simulink model "Wind_turbine_model_L"  (R2020a)
settings: Solver=daessc  StartTime=0.0  StopTime=70  RelTol=1e-3
model workspace (MAT data in the model file):
  Tw = Simulink.Parameter
  Tw.Value = [0; 0; 24.07; 18.74; 14.42; 10.93; 8.08; 5.74; 5.8; 4.17; 2.78; 1.59; 0.56; -0.34; -1.13; -1.83; -2.46; -3.02; -3.52; -3.98; -4.39; -3.77; -4.12; -4.43; -4.73]
  Tw.DataType = 'auto'
  Tw.Dimensions = [25 1]
  c = Simulink.Parameter
  c.Value = [3.65; 4.43; 4.56; 4.36; 4.03; 3.68; 3.35; 3.05; 2.79; 2.56; 2.37; 2.19; 2.04; 1.91; 1.79; 1.68; 1.59; 1.5; 1.43; 1.36; 1.29; 1.24; 1.18; 1.14; 1.09]
  c.DataType = 'auto'
  c.Dimensions = [25 1]
  r = Simulink.Parameter
  r.Value = [1.8; 3.6; 5.4; 7.2; 9; 10.8; 12.6; 14.4; 16.2; 18; 19.8; 21.6; 23.4; 25.2; 27; 28.8; 30.6; 32.4; 34.2; 36; 37.8; 39.6; 41.4; 43.2; 45]
  r.DataType = 'auto'
  r.Dimensions = [25 1]
values from neighbouring files (symbols this model uses):
  a1 = 0.5176    [data.mat]
  a2 = 116    [data.mat]
  a3 = 0.4    [data.mat]
  a4 = 5    [data.mat]
  a5 = 21    [data.mat]
  a6 = 0.0068    [data.mat]
  a7 = 0.09    [data.mat]
  a8 = 0.035    [data.mat]
  Ad = 6031.85789489    [data.mat]
  D = 1e-3    (= 0.001)    [Generator_specs.m]
  denp = den_P    [Wind_Turbine_Pitch.m]    (also in data.mat = [91260000000000 145900000000000 1.431e+17 7.554e+15 2.279e+1)
  dent = den_P    [Wind_Turbine_Pitch.m]    (also in data.mat = [91260000000000 145900000000000 1.431e+17 7.554e+15 2.279e+1)
  f = 50    [Generator_specs.m]
  Fs = Vs*sqrt(2/3)/(2*pi*f)    [Generator_specs.m]
  fsw = 4e3    (= 4000)    [Generator_specs.m]
  J = 127/2    (= 63.5)    [Generator_specs.m]
  ki_id = (wn1^2)*Lr*sigma    (= 491.599501999)    [Generator_specs.m]
  ki_n = ((wnn^2)*J)/p    (= 203200)    [Generator_specs.m]
  Kopt = ((0.5*ro*pi*(Radius^5)*cp_max)/(lambda_opt^3))    (= 227539.221001)    [Generator_specs.m]
  kp_id = (2*wn1*sigma*Lr)-Rr    (= 0.5771)    [Generator_specs.m]
  kp_n = (2*wnn*J)/p    (= 5080)    [Generator_specs.m]
  Lm = 2.5e-3    (= 0.0025)    [Generator_specs.m]
  Lr = Lm + Lsi    (= 0.002587)    [Generator_specs.m]
  Ls = Lm + Lsi    (= 0.002587)    [Generator_specs.m]
  Lsi = 0.087e-3    (= 8.7e-05)    [Generator_specs.m]
  N = 100    [Generator_specs.m]
  nump = num_P    [Wind_Turbine_Pitch.m]    (also in data.mat = [16590000 26450000 25540000000 6335000000 3680000000000])
  numt = num_T    [Wind_Turbine_Pitch.m]    (also in data.mat = [-75000000 -527900000000 -306700000000000])
  p = 2    [Generator_specs.m]
  Ps = 2e6    (= 2000000)    [Generator_specs.m]
  Rr = 2.9e-3    (= 0.0029)    [Generator_specs.m]
  Rs = 2.6e-3    (= 0.0026)    [Generator_specs.m]
  s = tf('s')    [Wind_Turbine_Pitch.m]
  sigma = 1 - Lm^2/(Ls*Lr)    (= 0.0661284179513)    [Generator_specs.m]    (also in data.mat = 0.075)
  Tem = 12732    [Generator_specs.m]
  Tgd_max = 14000    [Wind_Turbine_Pitch.m]    (also in data.mat)
  Tie = 1    [data.mat]
  Tiu = 10000    [data.mat]
  Tix = 1    [data.mat]
  Tpe = 1    [data.mat]
  Tpu = 10000    [data.mat]
  Tpx = 10000    [data.mat]
  Ts = 1/fsw/50    (= 5e-06)    [Generator_specs.m]
  Vbus = Vr_stator*sqrt(2)    [Generator_specs.m]
  Vs = 690    [Generator_specs.m]
  WT_Params =     [data.mat]
undefined symbols (not defined in the file or in its folder): DiscIntNeverNeededParam, sigbuilder_block, X, Y, Z
libraries: sm_lib x21, fl_lib x18, nesl_utility x18, powerlib x8, sdl_lib x3, powerlib_meascontrol x1
(part 1 of 3)
settings Model: Creator=param  LastModifiedBy=param
settings SolverCC: ZeroCrossControl=DisableAll  ZeroCrossAlgorithm=Adaptive
settings ModelReferenceCC: EnableParallelModelReferenceBuilds=on  ModelReferenceMinAlgLoopOccurrences=on

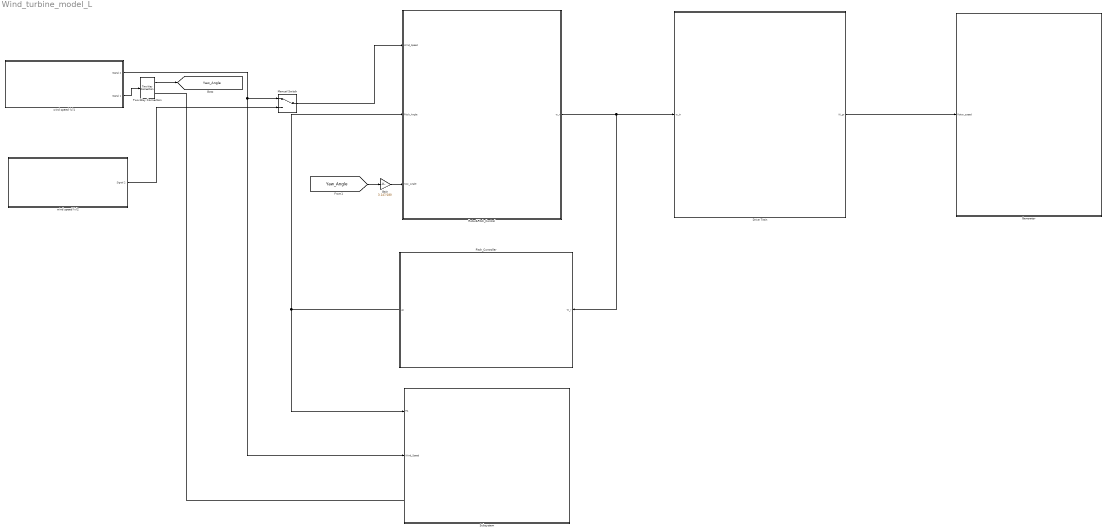
== system Wind_turbine_model_L ==
  Drive Train : Subsystem
  Gain : Gain  Gain=3.147/180
  Generator : Subsystem
  Manual Switch : ManualSwitch
  Pitch_Controller : Subsystem
  Rotor&Pitch_Control : Subsystem
  Subsystem : Subsystem
  Two-Way Connection : TwoWayConnection
  wind speed (v)1 : Subsystem  Tag=STV Subsys  LoadFcn=sigbuilder_block('load');  StartFcn=sigbuilder_block('start');  StopFcn=sigbuilder_block('stop');  ClipboardFcn=sigbuilder_block('clipboard');  mask(Sigbuilder block){tuvar=[0:10]}
      mask help: Simulink:masks:SigbuilderBlock_MD
      mask init:
      | if ~strcmp(get_param(bdroot(gcbh),'SimulationStatus'),'stopped') tuvar = sigbuilder_block('maskInit'); end
      settings: CopyFcn=sigbuilder_block('copy');  DeleteFcn=sigbuilder_block('delete');  ModelCloseFcn=sigbuilder_block('modelClose');  PreSaveFcn=sigbuilder_block('preSave');  PauseFcn=sigbuilder_block('pause');  ContinueFcn=sigbuilder_block('continue');  NameChangeFcn=sigbuilder_block('namechange');  OpenFcn=sigbuilder_block('open',[6 0 1012.5 477.75 ]);  CloseFcn=sigbuilder_block('close');
      mask Display: plot(0, 0, 100, 100,[2, 2, 32, 32, 2], [68, 8, 8, 68, 68],[32, 2], [38, 38], [32, 19, 2],[53, 60, 44], [32, 17, 17, 2],[16, 16, 31, 31]);txt = getActiveGroup(gcbh);text(2, 100, txt,'verticalAlignment', 'top');
  wind speed (v)2 : Subsystem  Tag=STV Subsys  LoadFcn=sigbuilder_block('load');  StartFcn=sigbuilder_block('start');  StopFcn=sigbuilder_block('stop');  ClipboardFcn=sigbuilder_block('clipboard');  mask(Sigbuilder block){tuvar=[0:10]}
      mask help: Simulink:masks:SigbuilderBlock_MD
      mask init:
      | if ~strcmp(get_param(bdroot(gcbh),'SimulationStatus'),'stopped') tuvar = sigbuilder_block('maskInit'); end
      settings: CopyFcn=sigbuilder_block('copy');  DeleteFcn=sigbuilder_block('delete');  ModelCloseFcn=sigbuilder_block('modelClose');  PreSaveFcn=sigbuilder_block('preSave');  PauseFcn=sigbuilder_block('pause');  ContinueFcn=sigbuilder_block('continue');  NameChangeFcn=sigbuilder_block('namechange');  OpenFcn=sigbuilder_block('open',[289.8 114 442.2 307.8 ]);  CloseFcn=sigbuilder_block('close');
      mask Display: plot(0, 0, 100, 100,[2, 2, 32, 32, 2], [68, 8, 8, 68, 68],[32, 2], [38, 38], [32, 19, 2],[53, 60, 44], [32, 17, 17, 2],[16, 16, 31, 31]);txt = getActiveGroup(gcbh);text(2, 100, txt,'verticalAlignment', 'top');
  tag scope: Yaw_Angle=global
  wires:
  Drive Train/1(W_gr) -> Generator/1(Rotor_speed)
  Rotor&Pitch_Control/1(w_r) -> Pitch_Controller/1(W_r), Drive Train/1(w_tr)
  wind speed (v)2/1(Signal 2) -> Manual Switch/2
  Manual Switch/1 -> Rotor&Pitch_Control/1(Wind_Speed)
  wind speed (v)1/1(Signal 2) -> Manual Switch/1, Subsystem/2(Wind_Speed)
  wind speed (v)1/2(Signal 1) -> Two-Way Connection/1
  [Yaw_Angle] -> Gain/1
  Two-Way Connection/1 -> [Yaw_Angle]
  Gain/1 -> Rotor&Pitch_Control/3(Yaw_Angle)
  Pitch_Controller/1(up) -> Subsystem/1(PA), Rotor&Pitch_Control/2(Pitch_Angle)
  connections:
  Subsystem/LConn1 -- Two-Way Connection/RConn1

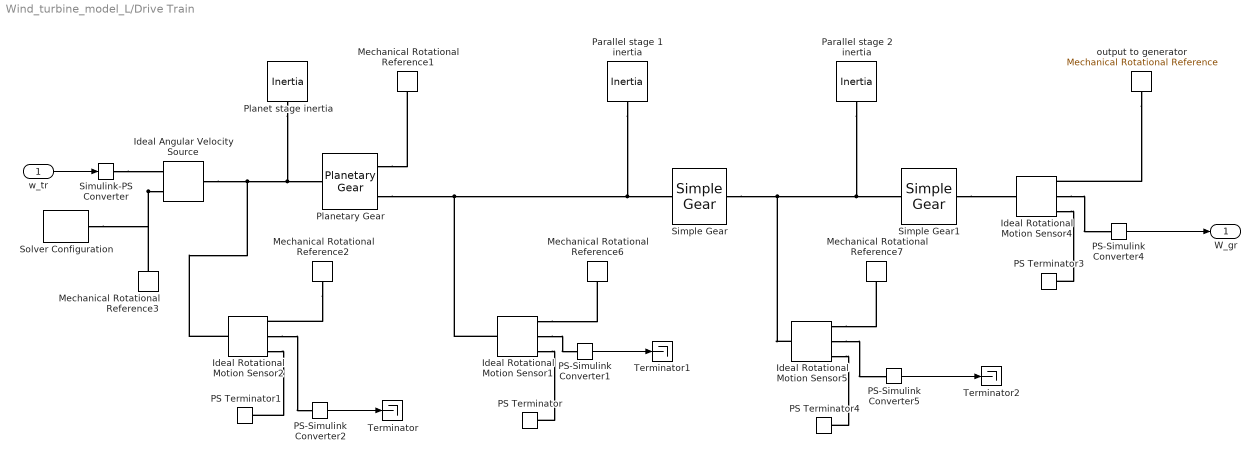
== system Wind_turbine_model_L/Drive Train ==
  w_tr : Inport
  Ideal Angular Velocity Source : fl_lib/Mechanical/Mechanical Sources/Ideal Angular Velocity Source
  Ideal Rotational Motion Sensor{1..2,4..5} (4 alike) : fl_lib/Mechanical/Mechanical Sensors/Ideal Rotational Motion Sensor  wrap_angle=simscape.enum.onoff.off  offset=0 rad
  Mechanical Rotational Reference{1..3,6..7} (5 alike) : fl_lib/Mechanical/Rotational Elements/Mechanical Rotational Reference
  PS Terminator{,1,3..4} (4 alike) : fl_lib/Physical Signals/Sinks/PS Terminator
  PS-Simulink Converter{1..2,4..5} (4 alike) : nesl_utility/PS-Simulink Converter  PhysicalDomain=network_engine_domain  SubClassName=ps_output  LeftPortType=input  RightPortType=output  PseudoPeriodic=off  Frequencies=[]  Unit=inherit  AffineConversion=off
  Parallel stage 1 inertia : fl_lib/Mechanical/Rotational Elements/Inertia  inertia=100 kg*m^2  w_specify=off  w_priority=High  w=0 rad/s  w_nominal_specify=off  w_nominal_unit=rad/s  w_nominal_value=1  t_specify=off  t_priority=None  t=0 N*m  t_nominal_specify=off  t_nominal_unit=N*m  t_nominal_value=1
  Parallel stage 2 inertia : fl_lib/Mechanical/Rotational Elements/Inertia  inertia=100 kg*m^2  w_specify=off  w_priority=High  w=0 rad/s  w_nominal_specify=off  w_nominal_unit=rad/s  w_nominal_value=1  t_specify=off  t_priority=None  t=0 N*m  t_nominal_specify=off  t_nominal_unit=N*m  t_nominal_value=1
  Planet stage inertia : fl_lib/Mechanical/Rotational Elements/Inertia  inertia=100 kg*m^2  w_specify=off  w_priority=High  w=0 rad/s  w_nominal_specify=off  w_nominal_unit=rad/s  w_nominal_value=1  t_specify=off  t_priority=None  t=0 N*m  t_nominal_specify=off  t_nominal_unit=N*m  t_nominal_value=1
  Planetary Gear : sdl_lib/Gears/Planetary Gear  rs_ratio=7  friction_model=sdl.enum.gear_friction.none  mu_visc=[0, 0] N*m/(rad/s)  efficiency=[.96, .98]  temperature_TLU=[280, 300, 320] K  efficiency_sp_TLU=[.95, .9, .85]  efficiency_rp_TLU=[.95, .9, .85]  pwr_thr=[.001, .001] W  thermal_mass=50 J/K  T_init=300 K  model_inertia=simscape.enum.onoff.off  planet_inertia=100 kg*m^2
      settings: SourceProductBaseCode=LD
  Simple Gear : sdl_lib/Gears/Simple Gear  ratio=1/4.5  rotation_direction=2  friction_model=sdl.enum.gear_efficiencies_load.off  T_noload=0.1 N*m  T_nom=5 N*m  efficiency_nom=0.8  efficiency=0.8  mu_visc=[0, 0] N*m/(rad/s)  w_thr=0.01 rad/s  pwr_thr=0.001 W  enable_faults=simscape.enum.onoff.off  efficiency_fault=0.05  external_fault=simscape.enum.onoff.off  temporal_fault=simscape.enum.onoff.off  fault_time=5 s  fault_angles=pi / 12 rad  report_fault=1  temperature_TLU=[280, 300, 320] K  load_TLU=[1, 5, 10] N*m  efficiency_TLU=[.95, .9, .85]  efficiency_TLU2=[.85, .8, .75; .95, .9, .85; .85, .8, .7]  thermal_mass=50 J/K  T_init=300 K
  Simple Gear1 : sdl_lib/Gears/Simple Gear  ratio=1/3.15  rotation_direction=2  friction_model=sdl.enum.gear_efficiencies_load.off  T_noload=0.1 N*m  T_nom=5 N*m  efficiency_nom=0.8  efficiency=0.8  mu_visc=[0, 0] N*m/(rad/s)  w_thr=0.01 rad/s  pwr_thr=0.001 W  enable_faults=simscape.enum.onoff.off  efficiency_fault=0.05  external_fault=simscape.enum.onoff.off  temporal_fault=simscape.enum.onoff.off  fault_time=5 s  fault_angles=pi / 12 rad  report_fault=1  temperature_TLU=[280, 300, 320] K  load_TLU=[1, 5, 10] N*m  efficiency_TLU=[.95, .9, .85]  efficiency_TLU2=[.85, .8, .75; .95, .9, .85; .85, .8, .7]  thermal_mass=50 J/K  T_init=300 K
  Simulink-PS Converter : nesl_utility/Simulink-PS Converter  PhysicalDomain=network_engine_domain  SubClassName=ps_input  LeftPortType=input  RightPortType=output  PseudoPeriodic=off  Frequencies=[]  NoiseDistribution=none  NoiseParameters=[]  Unit=1  AffineConversion=off  FilteringAndDerivatives=filter  SimscapeFilterOrder=2  InputFilterTimeConstant=0.001  UdotUserProvided=0
  Solver Configuration : nesl_utility/Solver Configuration  PhysicalDomain=network_engine_domain  SubClassName=solver  LeftPortType=input  RightPortType=generic  Tones=[]  Harmonics=[]  SimulateNoise=off  Profile=off  UseLocalSampling=off  EnableSwitchedLinearOptims=on  FrequencyDomain=off  UseCCode=off  RelTol=0.001  AbsTol=1e-06  MinStep=1e-09  ToWorkspace=off  RevertToSquareIcSolve=off  NumHomotopyIterations=100  PhasorMode=off  PhasorModeNumHarmonics=1  DoDC=off  ResidualTolerance=1e-09  UseLocalSolver=off  LocalSolverChoice=NE_BACKWARD_EULER_ADVANCER  LocalSolverSampleTime=0.001  DoFixedCost=off  MaxNonlinIter=3  MaxModeIter=2  LinearAlgebra=auto  EquationFormulation=NE_TIME_EF  DelaysMemoryBudget=1024  AutomaticFiltering=on  FilteringTimeConstant=0.001  PartitionStorageMethod=AS_NEEDED  PartitionMemoryBudget=1024  PartitionMethod=ROBUST
  Terminator : Terminator
  Terminator1 : Terminator
  Terminator2 : Terminator
  output to generator : fl_lib/Mechanical/Rotational Elements/Mechanical Rotational Reference
  W_gr : Outport
  wires:
  PS-Simulink Converter4/1 -> W_gr/1
  w_tr/1 -> Simulink-PS Converter/1
  PS-Simulink Converter2/1 -> Terminator/1
  PS-Simulink Converter1/1 -> Terminator1/1
  PS-Simulink Converter5/1 -> Terminator2/1
  connections:
  Ideal Angular Velocity Source/LConn1 -- Ideal Rotational Motion Sensor2/LConn1 -- Planet stage inertia/LConn1 -- Planetary Gear/LConn1
  Planetary Gear/RConn1 -- Mechanical Rotational Reference1/LConn1
  Ideal Angular Velocity Source/RConn2 -- Mechanical Rotational Reference3/LConn1 -- Solver Configuration/RConn1
  Ideal Rotational Motion Sensor1/RConn2 -- PS-Simulink Converter1/LConn1
  Ideal Rotational Motion Sensor5/RConn3 -- PS Terminator4/LConn1
  Planetary Gear/RConn2 -- Ideal Rotational Motion Sensor1/LConn1 -- Simple Gear/LConn1 -- Parallel stage 1 inertia/LConn1
  Ideal Rotational Motion Sensor1/RConn1 -- Mechanical Rotational Reference6/LConn1
  Mechanical Rotational Reference2/LConn1 -- Ideal Rotational Motion Sensor2/RConn1
  Ideal Rotational Motion Sensor4/RConn2 -- PS-Simulink Converter4/LConn1
  Ideal Rotational Motion Sensor5/RConn2 -- PS-Simulink Converter5/LConn1
  Ideal Rotational Motion Sensor2/RConn3 -- PS Terminator1/LConn1
  Simple Gear1/RConn1 -- Ideal Rotational Motion Sensor4/LConn1
  Simple Gear/RConn1 -- Ideal Rotational Motion Sensor5/LConn1 -- Parallel stage 2 inertia/LConn1 -- Simple Gear1/LConn1
  Ideal Rotational Motion Sensor4/RConn3 -- PS Terminator3/LConn1
  Ideal Rotational Motion Sensor5/RConn1 -- Mechanical Rotational Reference7/LConn1
  Ideal Rotational Motion Sensor2/RConn2 -- PS-Simulink Converter2/LConn1
  output to generator/LConn1 -- Ideal Rotational Motion Sensor4/RConn1
  Ideal Rotational Motion Sensor1/RConn3 -- PS Terminator/LConn1
  Simulink-PS Converter/RConn1 -- Ideal Angular Velocity Source/RConn1

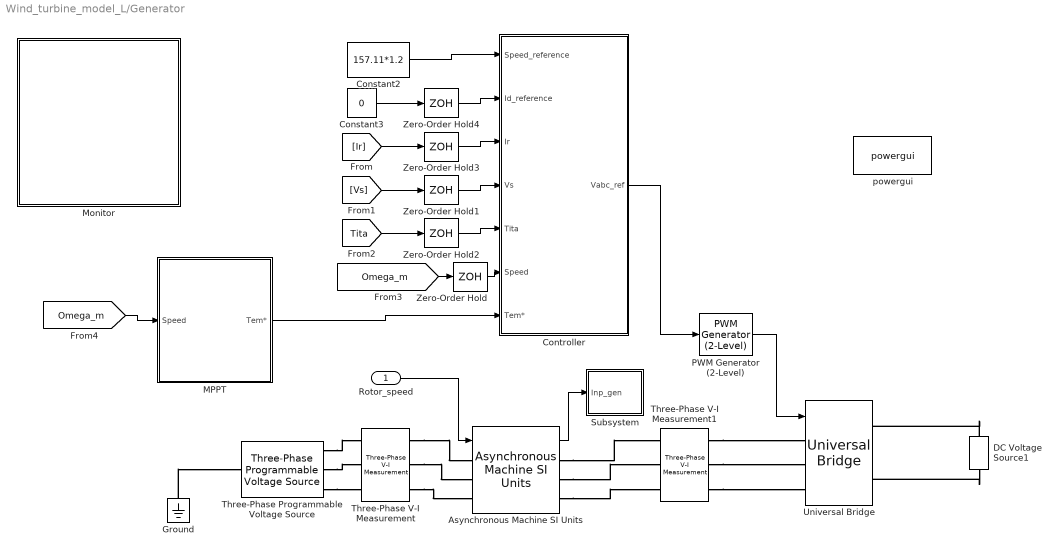
== system Wind_turbine_model_L/Generator ==
  Rotor_speed : Inport
  Asynchronous Machine SI Units : powerlib/Machines/Asynchronous Machine SI Units  RotorType=Wound  PresetModel=No  MechanicalLoad=Speed w  ShowDetailedParameters=on  ReferenceFrame=Rotor  Units=SI  MeasurementBus=off  NominalParameters=[Ps Vs f]  Stator=[Rs, Lsi]  Rotor=[Rr, Lsi]  Cage1=[0.4155 0.002066]  Cage2=[0.4168 0.0003495]  Lm=Lm  Mechanical=[J D 2]  PolePairs=2  InitialConditions=[1 0 0 0 0 0 0 0]  SimulateSaturation=off  Saturation=[14.03593122, 27.81365428, 53.79336849, 72.68890987, 97.98006896, 148.6815601, 215.7428561, 302.9841135, 428.7778367 ; 230, 322, 414, 460, 506, 552, 598, 644, 690]  LoadFlowParameters=1492000  TsPowergui=0  TsBlock=-1  IterativeModel=Trapezoidal non iterative  IterativeDiscreteModel=Trapezoidal non iterative  Pmec=1.492e+006
  Constant2 : Constant  Value=157.11*1.2
  Constant3 : Constant  Value=0
  Controller : Subsystem
  DC Voltage Source1 : powerlib/Electrical Sources/DC Voltage Source  Amplitude=Vbus  Measurements=None
  Ground : powerlib/Elements/Ground  LConnTagsString=a
  MPPT : Subsystem
  Monitor : Subsystem
  PWM Generator (2-Level) : powerlib_meascontrol/Pulse & Signal Generators/PWM Generator (2-Level)  ModulatorType=Three-phase bridge (6 pulses)  ModulatorMode=Unsynchronized  Fc=fsw  Pc=90  nF=27  MinMax="[ -1  1 ]"  SamplingTechnique=Symmetrical regular (single edge)  ModulatingSignals=off  m=0.8  Freq=60  Phase=0  Ts=0  ShowCarrierOutport=off
  Subsystem : Subsystem
  Three-Phase Programmable Voltage Source : powerlib/Electrical Sources/Three-Phase Programmable Voltage Source  PositiveSequence=[Vs 0 f]  VariationEntity=None  VariationType=Table of time-amplitude pairs  VariationTypeAlt=Step  VariationStep=0.5  VariationRate=10  VariationMagnitude=0.3  VariationFrequency=2  VariationTiming=[1 2]  VariationPhaseA=off  Amplitudes=[1 0.8 1.2 1.0]  TimeValues=[0 0.1 0.15 0.2]  HarmonicGeneration=off  HarmonicA=[3 0.2 -25 0]  HarmonicB=[2 0.15 35 2]  Timing="[0.05  3]"  BusType=swing  Pref=0  Qref=0  Qmin=-inf  Qmax=inf
  Three-Phase V-I Measurement : powerlib/Measurements/Three-Phase V-I Measurement  VoltageMeasurement=phase-to-ground  SetLabelV=on  LabelV=Vs  Vpu=on  VpuLL=off  CurrentMeasurement=yes  SetLabelI=on  LabelI=Is  Ipu=off  Pbase=100e6  Vbase=500e3  OutputType=Complex  PhasorSimulation=off  PSBequivalent=0
  Three-Phase V-I Measurement1 : powerlib/Measurements/Three-Phase V-I Measurement  VoltageMeasurement=no  SetLabelV=off  LabelV=Vr  Vpu=off  VpuLL=off  CurrentMeasurement=yes  SetLabelI=on  LabelI=Ir  Ipu=off  Pbase=100e6  Vbase=500e3  OutputType=Complex  PhasorSimulation=off  PSBequivalent=0
  Universal Bridge : powerlib/Power Electronics/Universal Bridge  Arms=3  SnubberResistance=1e5  SnubberCapacitance=inf  Device=Ideal Switches  Ron=1e-3  Lon=0  ForwardVoltages="[  0  0  ]"  ForwardVoltage=0  GTOparameters=[ 10e-6 , 20e-6 ]  IGBTparameters=[ 1e-6 , 2e-6 ]  Measurements=None  Measurements_2=None  converterType=Rectifier
  Zero-Order Hold{,1..4} (5 alike) : ZeroOrderHold  SampleTime=1/fsw
  powergui : powerlib/powergui  Priority=1  SimulationMode=Continuous  SampleTime=Ts  frequency=60  Iterations=50  frequencyindice=50  Pbase=100e6  ErrMax=1e-4  UnitsV=kV  UnitsW=MW  buscounter=0  FunctionMessages=off  echomessages=off  EnableUseOfTLC=off  CurrentSourceSwitches=off  DisableSnubberDevices=off  DisableRonSwitches=off  DisableVfSwitches=off  DisplayEquations=off  AutomaticDiscreteSolvers=off  SolverType=Tustin/Backward Euler (TBE)  Interpol=off  ExternalGateDelay=off  methode=off  Ts=100  x0status=blocks  SPID=on  SwTol=0  HookPort=off  NonlinearTolerance=1e-4  nMaxIteration=100  ContinueOnMaxIteration=off  RestoreLinks=warning  ResistiveCurrentMeasurement=off  Frange=[0:2:500]  Ylog=off  Xlog=on  ShowGrid=off  save=off  variable=ZData  structure=0  ZoomFFT=off  StartTime=0.0  cycles=1  DisplayStyle=1  fundamental=60  FreqAxis=off  MaxFrequency=1000  frequencyindicesteady=1  RmsSteady=1  display=off
  wires:
  Zero-Order Hold2/1 -> Controller/5(Tita)
  [Tita] -> Zero-Order Hold2/1
  Zero-Order Hold/1 -> Controller/6(Speed)
  [Vs] -> Zero-Order Hold1/1
  Zero-Order Hold4/1 -> Controller/2(Id_reference)
  Zero-Order Hold1/1 -> Controller/4(Vs)
  [Ir] -> Zero-Order Hold3/1
  Asynchronous Machine SI Units/1 -> Subsystem/1(Inp_gen)
  PWM Generator (2-Level)/1 -> Universal Bridge/1
  Constant2/1 -> Controller/1(Speed_reference)
  Constant3/1 -> Zero-Order Hold4/1
  [Omega_m] -> Zero-Order Hold/1
  Zero-Order Hold3/1 -> Controller/3(Ir)
  Controller/1(Vabc_ref) -> PWM Generator (2-Level)/1
  Rotor_speed/1 -> Asynchronous Machine SI Units/1
  [Omega_m] -> MPPT/1(Speed)
  MPPT/1(Tem*) -> Controller/7(Tem*)
  connections:
  Three-Phase V-I Measurement1/LConn3 -- Universal Bridge/LConn3
  Asynchronous Machine SI Units/RConn1 -- Three-Phase V-I Measurement1/RConn1
  Three-Phase V-I Measurement/RConn1 -- Asynchronous Machine SI Units/LConn1
  DC Voltage Source1/LConn1 -- Universal Bridge/RConn2
  Three-Phase Programmable Voltage Source/RConn3 -- Three-Phase V-I Measurement/LConn3
  Three-Phase V-I Measurement1/LConn2 -- Universal Bridge/LConn2
  Three-Phase Programmable Voltage Source/RConn2 -- Three-Phase V-I Measurement/LConn2
  Three-Phase Programmable Voltage Source/RConn1 -- Three-Phase V-I Measurement/LConn1
  Three-Phase V-I Measurement1/LConn1 -- Universal Bridge/LConn1
  Three-Phase V-I Measurement/RConn2 -- Asynchronous Machine SI Units/LConn2
  Three-Phase V-I Measurement/RConn3 -- Asynchronous Machine SI Units/LConn3
  Asynchronous Machine SI Units/RConn3 -- Three-Phase V-I Measurement1/RConn3
  Ground/LConn1 -- Three-Phase Programmable Voltage Source/LConn1
  DC Voltage Source1/RConn1 -- Universal Bridge/RConn1
  Asynchronous Machine SI Units/RConn2 -- Three-Phase V-I Measurement1/RConn2

== system Wind_turbine_model_L/Pitch_Controller ==
  note: um
  note: Wref
  W_r : Inport
  Controller : Subsystem
  Reference : TransferFcn  Denominator=[1 1]
  Step : Step  Time=0  After=1.8  SampleTime=0
  Sum3 : Sum  Inputs=|+-
  up : Outport
  wires:
  W_r/1 -> Sum3/2
  Step/1 -> Controller/2(um), Reference/1
  Reference/1 -> Sum3/1, Controller/1(xm)
  Sum3/1 -> Controller/3(ey)
  Controller/1(up) -> up/1

== system Wind_turbine_model_L/Rotor&Pitch_Control ==
  Wind_Speed : Inport
  Pitch_Angle : Inport  Port=2
  Yaw_Angle : Inport  Port=3
  Abs : Abs
  Constant : Constant  Value=Tgd_max
  From : From  Commented=on  GotoTag=Tem_ref
  Wr Plant : Subsystem
  w_r : Outport
  wires:
  Wr Plant/1(Wr(s)) -> w_r/1
  Wind_Speed/1 -> Wr Plant/1(v(s))
  Abs/1 -> Wr Plant/3(Tgd(s))
  Pitch_Angle/1 -> Wr Plant/2(Betad(s))
  Yaw_Angle/1 -> Wr Plant/4(Yaw_Angle)
  Constant/1 -> Abs/1

== system Wind_turbine_model_L/Subsystem ==
  PA : Inport
  Wind_Speed : Inport  Port=2
  Subsystem1 : Subsystem
  Yaw Controller : Subsystem
  Yaw Ctrl Scopes : Subsystem
  Yaw Angle : PMIOPort  Side=Left
  wires:
  Wind_Speed/1 -> Subsystem1/1(Wind_Speed)
  PA/1 -> Subsystem1/2(PA)
  connections:
  Yaw Angle/RConn1 -- Yaw Controller/LConn1
  Subsystem1/LConn1 -- Yaw Controller/RConn1

== system Wind_turbine_model_L/wind speed (v)1 ==
  Demux : Demux  Tag=STV Demux  Outputs=2
      settings: DisplayOption=none
  FromWs : FromWorkspace  Tag=STV FromWs  VariableName=tuvar
      SigBuilderData=|
      | common.afterFinalStr = 'Extrapolate'
      | common.sampleTime = 0
      | dataSet(1).timeRange = [0 120]
      | dataSet(1).name = 'Group 1'
      | dataSet(2).timeRange = [0 70]
      | dataSet(2).name = 'Group 2'
      | sbobj.Groups(1).Name = 'Group 1'
      | sbobj.Groups(1).Signals(1).Name = 'Signal 2'
      | sbobj.Groups(1).Signals(1).XData = [0 0.1 0.2 0.3 0.4 0.5 0.6 0.7 0.8 0.9 1 1.1 ... (1201 elements, 1x1201)]
      | sbobj.Groups(1).Signals(1).YData = [15.5376671395 16.8338850146 12.741153139 15.8621733204 15.3187652399 13.6923117037 14.5664079777 15.3426244665 18.5783969397 17.7694370299 13.6501130598 18.0349234663 ... (1201 elements, 1x1201)]
      | sbobj.Groups(1).Signals(2).Name = 'Signal 1'
      | sbobj.Groups(1).Signals(2).XData = [0 10 120]
      | sbobj.Groups(1).Signals(2).YData = [6.19231170369 7.06640797769 7.06640797769]
      | sbobj.Groups(1).TimeRange = [0 120]
      | sbobj.Groups(2).Name = 'Group 2'
      | sbobj.Groups(2).Signals(1).Name = 'Signal 2'
      | sbobj.Groups(2).Signals(1).XData = [0 2 4 6 8 70]
      | sbobj.Groups(2).Signals(1).YData = [15.2036737857 20.7 12.9 20.8 19.2 19.2]
      | sbobj.Groups(2).Signals(2).Name = 'Signal 1'
      | sbobj.Groups(2).Signals(2).XData = [0 1 21 31 36.6 54.8 70]
      | sbobj.Groups(2).Signals(2).YData = [0 0 0.45 0.5 1.17 0 0]
      | sbobj.Groups(2).TimeRange = [0 70]
  Signal 2 : Outport  Tag=STV Outport
  Signal 1 : Outport  Tag=STV Outport  Port=2
  wires:
  Demux/1 -> Signal 2/1
  FromWs/1 -> Demux/1
  Demux/2 -> Signal 1/1

== system Wind_turbine_model_L/wind speed (v)2 ==
  Demux : Demux  Tag=STV Demux  Outputs=1
      settings: DisplayOption=none
  FromWs : FromWorkspace  Tag=STV FromWs  VariableName=tuvar
      SigBuilderData=|
      | common.afterFinalStr = 'Extrapolate'
      | common.sampleTime = 0
      | dataSet(1).timeRange = [0 120]
      | dataSet(1).name = 'Group 1'
      | dataSet(2).timeRange = [0 120]
      | dataSet(2).name = 'Group 2'
      | sbobj.Groups(1).Name = 'Group 1'
      | sbobj.Groups(1).Signals.Name = 'Signal 2'
      | sbobj.Groups(1).Signals.XData = [0 0.1 0.2 0.3 0.4 0.5 0.6 0.7 0.8 0.9 1 1.1 ... (1201 elements, 1x1201)]
      | sbobj.Groups(1).Signals.YData = [15.5376671395 16.8338850146 12.741153139 15.8621733204 15.3187652399 13.6923117037 14.5664079777 15.3426244665 18.5783969397 17.7694370299 13.6501130598 18.0349234663 ... (1201 elements, 1x1201)]
      | sbobj.Groups(1).TimeRange = [0 120]
      | sbobj.Groups(2).Name = 'Group 2'
      | sbobj.Groups(2).Signals.Name = 'Signal 2'
      | sbobj.Groups(2).Signals.XData = [0 0.1 0.2 0.3 0.4 0.5 0.6 0.7 0.8 0.9 1 1.1 ... (1201 elements, 1x1201)]
      | sbobj.Groups(2).Signals.YData = [4.38462340739 6.13281595539 7.68524893308 14.1567938795 12.5388740598 4.30022611969 13.0698469327 8.45080844989 6.87389025362 8.42948580765 6.5900678834 6.75171130357 ... (1201 elements, 1x1201)]
      | sbobj.Groups(2).TimeRange = [0 120]
  Signal 2 : Outport  Tag=STV Outport
  wires:
  Demux/1 -> Signal 2/1
  FromWs/1 -> Demux/1

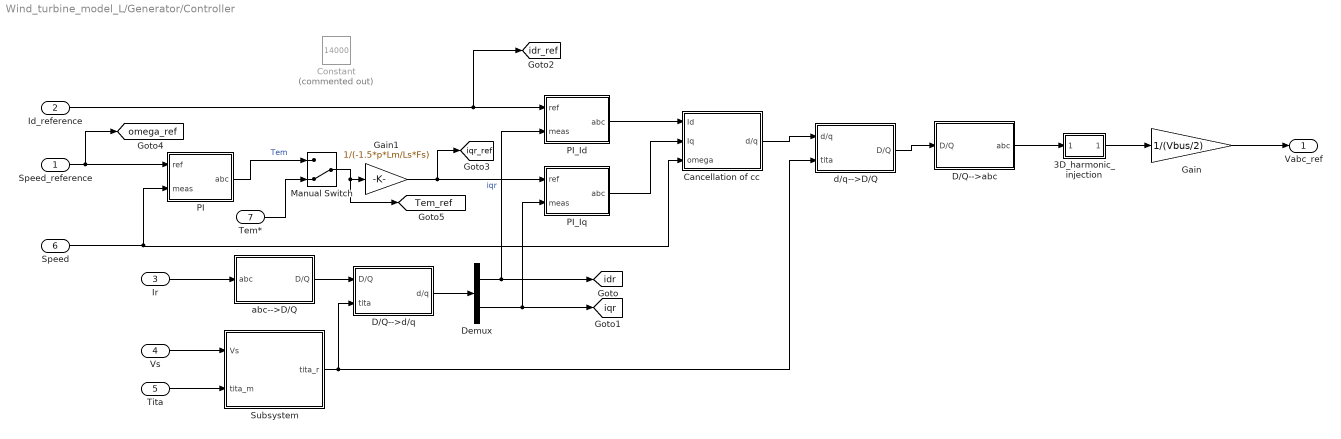
== system Wind_turbine_model_L/Generator/Controller ==
  Speed_reference : Inport
  Id_reference : Inport  Port=2
  Ir : Inport  Port=3
  Vs : Inport  Port=4
  Tita : Inport  Port=5
  Speed : Inport  Port=6
  Tem* : Inport  Port=7
  3D_harmonic_injection : Subsystem
  Cancellation of cc : Subsystem
  Constant : Constant  Commented=on  Value=14000
  D/Q-->abc : Subsystem
  D/Q-->d/q : Subsystem
  Demux : Demux  Outputs=2
  Gain : Gain  Gain=1/(Vbus/2)
  Gain1 : Gain  Gain=1/(-1.5*p*Lm/Ls*Fs)
  Manual Switch : ManualSwitch  CurrentSetting=0
  PI : Subsystem
  PI_Id : Subsystem
  PI_Iq : Subsystem
  Subsystem : Subsystem
  abc-->D/Q : Subsystem
  d/q-->D/Q : Subsystem
  Vabc_ref : Outport
  tag scope: Tem_ref=global, idr=global, idr_ref=global, iqr=global, iqr_ref=global, omega_ref=global
  wires:
  Id_reference/1 -> PI_Id/1(ref), [idr_ref]
  Gain1/1 -> PI_Iq/1(ref), [iqr_ref]  "iqr"
  Speed_reference/1 -> PI/1(ref), [omega_ref]
  Cancellation of cc/1(d/q) -> d/q-->D/Q/1(d/q)
  PI_Iq/1(abc) -> Cancellation of cc/2(Iq)
  PI_Id/1(abc) -> Cancellation of cc/1(Id)
  Demux/2 -> [iqr], PI_Iq/2(meas)
  Demux/1 -> [idr], PI_Id/2(meas)
  D/Q-->d/q/1(d/q) -> Demux/1
  Speed/1 -> Cancellation of cc/3(omega), PI/2(meas)
  Tita/1 -> Subsystem/2(tita_m)
  Vs/1 -> Subsystem/1(Vs)
  Subsystem/1(tita_r) -> D/Q-->d/q/2(tita), d/q-->D/Q/2(tita)
  3D_harmonic_injection/1(out1) -> Gain/1
  Ir/1 -> abc-->D/Q/1(abc)
  abc-->D/Q/1(D/Q) -> D/Q-->d/q/1(D/Q)
  d/q-->D/Q/1(D/Q) -> D/Q-->abc/1(D/Q)
  Gain/1 -> Vabc_ref/1
  D/Q-->abc/1(abc) -> 3D_harmonic_injection/1(ln1)
  PI/1(abc) -> Manual Switch/1  "Tem"
  Manual Switch/1 -> [Tem_ref], Gain1/1
  Tem*/1 -> Manual Switch/2

== system Wind_turbine_model_L/Generator/MPPT ==
  Speed : Inport
  Gain : Gain  Gain=1/N
  Gain1 : Gain  Gain=-Kopt
  Gain2 : Gain  Gain=1/N
  Square : Math  Operator=square  SaturateOnIntegerOverflow=on
  Tem* : Outport
  wires:
  Speed/1 -> Gain/1
  Gain/1 -> Square/1
  Square/1 -> Gain1/1
  Gain1/1 -> Gain2/1
  Gain2/1 -> Tem*/1

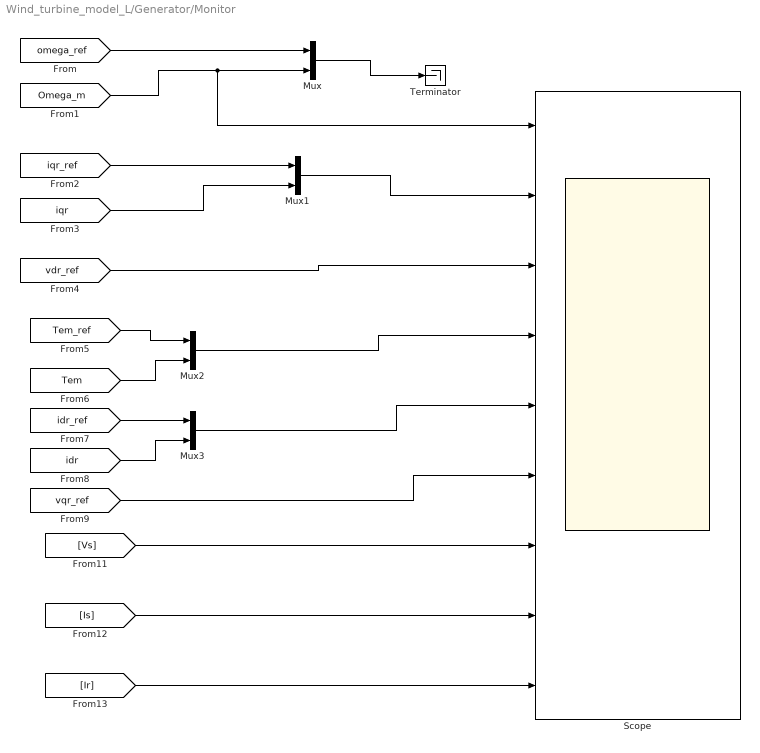
== system Wind_turbine_model_L/Generator/Monitor ==
  Mux{,1..3} (4 alike) : Mux  Inputs=2
  Scope : Scope  NumInputPorts=9
  Terminator : Terminator
  wires:
  [Ir] -> Scope/9
  [Is] -> Scope/8
  [Vs] -> Scope/7
  [vqr_ref] -> Scope/6
  Mux3/1 -> Scope/5
  Mux2/1 -> Scope/4
  [vdr_ref] -> Scope/3
  Mux1/1 -> Scope/2
  [idr] -> Mux3/2
  [idr_ref] -> Mux3/1
  [Tem] -> Mux2/2
  [Tem_ref] -> Mux2/1
  [iqr] -> Mux1/2
  [iqr_ref] -> Mux1/1
  [Omega_m] -> Scope/1, Mux/2
  [omega_ref] -> Mux/1
  Mux/1 -> Terminator/1

== system Wind_turbine_model_L/Generator/Subsystem ==
  Inp_gen : Inport
  Bus Selector : BusSelector  OutputSignals=Mechanical.Rotor angle thetam (rad),Mechanical.Rotor speed (wm),Mechanical.Electromagnetic torque Te (N*m)
  tag scope: Omega_m=global, Tem=global, Tita=global
  wires:
  Bus Selector/3 -> [Tem]  "<Electromagnetic torque Te (N*m)>"
  Bus Selector/2 -> [Omega_m]  "<Rotor speed (wm)>"
  Bus Selector/1 -> [Tita]  "<Rotor angle thetam (rad)>"
  Inp_gen/1 -> Bus Selector/1

== system Wind_turbine_model_L/Pitch_Controller/Controller ==
  xm : Inport
  um : Inport  Port=2
  ey : Inport  Port=3
  Ke : Subsystem
  Ke*ey : Product
  Ku : Subsystem
  Ku*um : Product
  Kx : Subsystem
  Kx*xm : Product
  Subtract : Sum  Inputs=+++
  up : Outport
  wires:
  Kx/1(Kx) -> Kx*xm/2
  Ke/1(Ke) -> Ke*ey/1
  Ku*um/1 -> Subtract/2
  Kx*xm/1 -> Subtract/1
  xm/1 -> Kx*xm/1, Kx/2(xm)
  ey/1 -> Kx/1(ey), Ku/1(ey), Ke*ey/2, Ke/1(ey)
  Ku/1(Ku) -> Ku*um/1
  Ke*ey/1 -> Subtract/3
  um/1 -> Ku/2(um), Ku*um/2
  Subtract/1 -> up/1

== system Wind_turbine_model_L/Rotor&Pitch_Control/Wr Plant ==
  note: yp
  note: Tg(s)
  v(s) : Inport
  Betad(s) : Inport  Port=2
  Tgd(s) : Inport  Port=3
  Yaw_Angle : Inport  Port=4
  GTg(s) : TransferFcn  Numerator=numt  Denominator=dent
  GTr(s) : TransferFcn  Numerator=nump  Denominator=denp
  Sum : Sum
  Wind Turbine : Subsystem  AncestorBlock=re_lib/Wind Generation/Wind Turbine  DialogController=POWERSYS.PowerSysDialog  mask(Wind Turbine){Pnom=2e6, Pelec_base=2e6/0.9, wind_base=9, P_wind_base=0.73, speed_nom=1.2, pitch_angle=10, c1_c6=[0.51763          116          0.4            5           21     0.006795], cp_nom=0.48, lambda_nom=8.1}
      mask prompts: Pnom "Nominal mechanical output power (W):"; Pelec_base "Base power of the electrical generator (VA):"; wind_base "Base wind speed (m/s):"; P_wind_base "Maximum power at base wind speed (pu of nominal mechanical power):"; speed_nom "Base rotational speed (p.u. of base generator speed):"; pitch_angle "Pitch angle beta to display wind-turbine power characteristics (beta >=0)  (deg):"
      mask help:
      | This block implements a variable pitch wind turbine model. The performance coefficient Cp of the turbine is the mechanical output power of the turbine divided by wind power and a function of wind speed, rotational speed, and pitch angle (beta). Cp reaches its maximum value at zero beta. Select the wind-turbine power characteristics display to plot the turbine characteristics at the specified pitch angle.
      |
      | The first input is the generator speed in per unit of the generator base speed. For a synchronous or asynchronous generator, the base speed is the synchronous speed. For a permanent-magnet generator, the base speed is defined as the speed producing nominal voltage at  no load. The second input is the blade pitch angle (beta) in degrees. The third input is the wind speed in m/s.
      |
      | The output is the torque applied to the generator shaft in per unit of the generator ratings.
      |
      | The turbine inertia must be added to the generator inertia.
      mask init:
      | c1=c1_c6(1);c2=c1_c6(2);c3=c1_c6(3);c4=c1_c6(4);c5=c1_c6(5);c6=c1_c6(6);
      | power_initmask();
      mask Help: helpview(psbhelp);
      mask DialogControl DisplayTurbChar Prompt: Display wind turbine power characteristics
      mask DialogControl DisplayTurbChar Callback: WindTurbinePlot(gcb)
      mask Display: disp('');
  Wr(s) : Outport
  wires:
  v(s)/1 -> Wind Turbine/3(v(s))
  Sum/1 -> Wind Turbine/1(Wr(s)), Wr(s)/1
  Tgd(s)/1 -> GTg(s)/1
  GTg(s)/1 -> Sum/2
  GTr(s)/1 -> Sum/1
  Betad(s)/1 -> Wind Turbine/2(Beta(s))
  Wind Turbine/1(Tr(s)) -> GTr(s)/1
  Yaw_Angle/1 -> Wind Turbine/4(Yaw_Angle)

== system Wind_turbine_model_L/Subsystem/Subsystem1 ==
  Wind_Speed : Inport
  PA : Inport  Port=2
  Aerodynamics : Subsystem
  Gain : Gain  Gain=1/200*(3.147/180)
  MultiBody_Blades : Subsystem
  Nacelle : Subsystem
  Subsystem : Subsystem
  Tower : Subsystem
  YC : PMIOPort  Side=Left
  wires:
  Wind_Speed/1 -> Aerodynamics/1(Wind speed)
  PA/1 -> Gain/1
  Gain/1 -> MultiBody_Blades/1(PA)
  connections:
  MultiBody_Blades/RConn2 -- Subsystem/LConn2
  MultiBody_Blades/RConn3 -- Subsystem/LConn3
  Subsystem/LConn4 -- Aerodynamics/RConn1
  Tower/RConn1 -- Nacelle/LConn2
  Nacelle/LConn1 -- Subsystem/RConn1
  MultiBody_Blades/RConn1 -- Subsystem/LConn1
  YC/RConn1 -- Nacelle/LConn3

== system Wind_turbine_model_L/Subsystem/Yaw Controller ==
  Demux : Demux  Outputs=[4 1]
  Selector : Selector  InputPortWidth=4  IndexOptions=Index vector (dialog)  Indices=[1 ]  OutputSizes=1
  Two-Way Connection : TwoWayConnection
  Two-Way Connection1 : TwoWayConnection
  Yaw Controller : Subsystem
  Y : PMIOPort  Tag=PMCPort  Side=Right
  M : PMIOPort  Tag=PMCPort  Port=2  Side=Left
  tag scope: Nacelle_Yaw_Rate=global, Yaw_Torque_Command=global
  wires:
  Selector/1 -> Two-Way Connection1/1
  Two-Way Connection1/1 -> Yaw Controller/1(Yaw Command)
  Demux/2 -> Yaw Controller/2(Yaw Rate), [Nacelle_Yaw_Rate]
  Demux/1 -> Selector/1, Yaw Controller/3(Yaw)
  Two-Way Connection/1 -> Demux/1
  Yaw Controller/1(Torque Command) -> [Yaw_Torque_Command], Two-Way Connection/1
  connections:
  Y/RConn1 -- Two-Way Connection/RConn1
  M/RConn1 -- Two-Way Connection1/RConn1

== system Wind_turbine_model_L/Subsystem/Yaw Ctrl Scopes ==
  Mux1 : Mux  Inputs=2
  Nacelle Yaw : Scope
  wires:
  Mux1/1 -> Nacelle Yaw/1  "Nacelle Yaw(deg)"
  [Yaw_Command] -> Mux1/2
  [Yaw_Angle] -> Mux1/1  "Nacelle_Yaw_Angle"

== system Wind_turbine_model_L/Generator/Controller/3D_harmonic_injection ==
  ln1 : Inport
  Gain : Gain  Gain=-0.5
  Max : MinMax  Function=max
  Min : MinMax
  Sum : Sum  Inputs=|++
  Sum1 : Sum  Inputs=|++
  out1 : Outport
  wires:
  Sum1/1 -> out1/1
  ln1/1 -> Sum1/1, Min/1, Max/1
  Gain/1 -> Sum1/2
  Max/1 -> Sum/2
  Min/1 -> Sum/1
  Sum/1 -> Gain/1

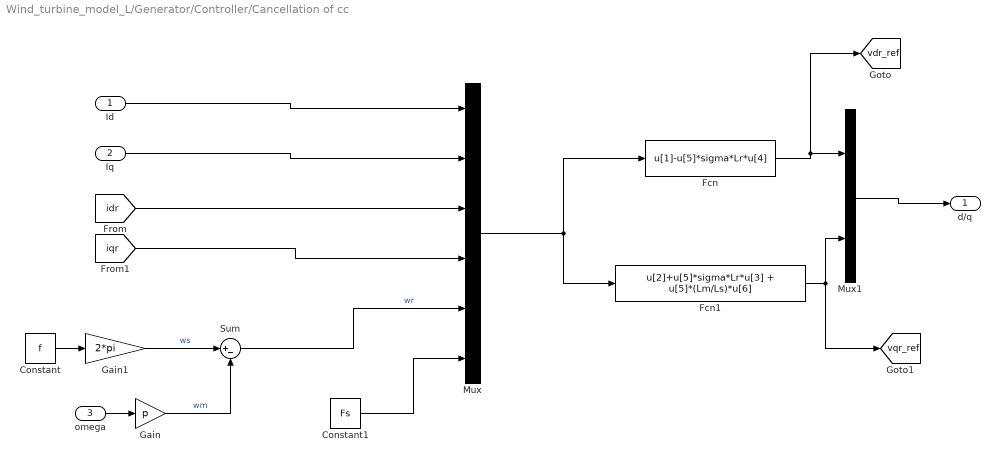
== system Wind_turbine_model_L/Generator/Controller/Cancellation of cc ==
  Id : Inport
  Iq : Inport  Port=2
  omega : Inport  Port=3
  Constant : Constant  Value=f
  Constant1 : Constant  Value=Fs
  Fcn : Fcn  Expr=u[1]-u[5]*sigma*Lr*u[4]
  Fcn1 : Fcn  Expr=u[2]+u[5]*sigma*Lr*u[3] + u[5]*(Lm/Ls)*u[6]
  Gain : Gain  Gain=p
  Gain1 : Gain  Gain=2*pi
  Mux : Mux  Inputs=6
  Mux1 : Mux  Inputs=2
  Sum : Sum  Inputs=|+-
  d/q : Outport
  tag scope: vdr_ref=global, vqr_ref=global
  wires:
  Mux1/1 -> d/q/1
  Fcn1/1 -> Mux1/2, [vqr_ref]
  Fcn/1 -> Mux1/1, [vdr_ref]
  Mux/1 -> Fcn/1, Fcn1/1
  Constant1/1 -> Mux/6
  Sum/1 -> Mux/5  "wr"
  [iqr] -> Mux/4
  [idr] -> Mux/3
  Iq/1 -> Mux/2
  Id/1 -> Mux/1
  Gain/1 -> Sum/2  "wm"
  Gain1/1 -> Sum/1  "ws"
  Constant/1 -> Gain1/1
  omega/1 -> Gain/1

== system Wind_turbine_model_L/Generator/Controller/D//Q-->abc ==
  D/Q : Inport
  Fcn : Fcn  Expr=u[1]
  Fcn1 : Fcn  Expr=-(u[1]/2) + u[2]*(sqrt(3)/2)
  Fcn2 : Fcn  Expr=-(u[1]/2) - u[2]*(sqrt(3)/2)
  Mux : Mux  Inputs=3
  abc : Outport
  wires:
  Mux/1 -> abc/1
  Fcn2/1 -> Mux/3
  Fcn1/1 -> Mux/2
  Fcn/1 -> Mux/1
  D/Q/1 -> Fcn/1, Fcn1/1, Fcn2/1

== system Wind_turbine_model_L/Generator/Controller/D//Q-->d//q ==
  D/Q : Inport
  tita : Inport  Port=2
  Fcn : Fcn  Expr=u[1]*cos(u[3])+u[2]*sin(u[3])
  Fcn1 : Fcn  Expr=-u[1]*sin(u[3]) + u[2]*cos(u[3])
  Mux : Mux  Inputs=2
  Mux1 : Mux  Inputs=2
  d/q : Outport
  wires:
  Mux1/1 -> Fcn1/1, Fcn/1
  tita/1 -> Mux1/2
  D/Q/1 -> Mux1/1
  Mux/1 -> d/q/1
  Fcn1/1 -> Mux/2
  Fcn/1 -> Mux/1

== system Wind_turbine_model_L/Generator/Controller/PI ==
  ref : Inport
  meas : Inport  Port=2
  Discrete-Time Integrator : DiscreteIntegrator  SampleTime=1/fsw  LimitOutput=on  UpperSaturationLimit=Tem  LowerSaturationLimit=-Tem  ICPrevOutput=DiscIntNeverNeededParam  ICPrevScaledInput=DiscIntNeverNeededParam
  Gain : Gain  Gain=kp_n
  Gain1 : Gain  Gain=ki_n
  Saturation : Saturate  UpperLimit=Tem  LowerLimit=-Tem
  Sum : Sum  Inputs=|+-
  Sum1 : Sum  Inputs=|++
  abc : Outport
  wires:
  Saturation/1 -> abc/1
  Discrete-Time Integrator/1 -> Sum1/2
  Sum1/1 -> Saturation/1
  Gain/1 -> Sum1/1
  Gain1/1 -> Discrete-Time Integrator/1
  Sum/1 -> Gain/1, Gain1/1
  meas/1 -> Sum/2
  ref/1 -> Sum/1

== system Wind_turbine_model_L/Generator/Controller/PI_Id ==
  ref : Inport
  meas : Inport  Port=2
  Discrete-Time Integrator : DiscreteIntegrator  SampleTime=1/fsw  LimitOutput=on  UpperSaturationLimit=Vbus/sqrt(3)  LowerSaturationLimit=-Vbus/sqrt(3)  ICPrevOutput=DiscIntNeverNeededParam  ICPrevScaledInput=DiscIntNeverNeededParam
  Gain : Gain  Gain=kp_id
  Gain1 : Gain  Gain=ki_id
  Saturation : Saturate  UpperLimit=Vbus/sqrt(3)  LowerLimit=-Vbus/sqrt(3)
  Sum : Sum  Inputs=|+-
  Sum1 : Sum  Inputs=|++
  abc : Outport
  wires:
  Saturation/1 -> abc/1
  Discrete-Time Integrator/1 -> Sum1/2
  Sum1/1 -> Saturation/1
  Gain/1 -> Sum1/1
  Gain1/1 -> Discrete-Time Integrator/1
  Sum/1 -> Gain/1, Gain1/1
  meas/1 -> Sum/2
  ref/1 -> Sum/1

== system Wind_turbine_model_L/Generator/Controller/PI_Iq ==
  ref : Inport
  meas : Inport  Port=2
  Discrete-Time Integrator : DiscreteIntegrator  SampleTime=1/fsw  LimitOutput=on  UpperSaturationLimit=Vbus/sqrt(3)  LowerSaturationLimit=-Vbus/sqrt(3)  ICPrevOutput=DiscIntNeverNeededParam  ICPrevScaledInput=DiscIntNeverNeededParam
  Gain : Gain  Gain=kp_id
  Gain1 : Gain  Gain=ki_id
  Saturation : Saturate  UpperLimit=Vbus/sqrt(3)  LowerLimit=-Vbus/sqrt(3)
  Sum : Sum  Inputs=|+-
  Sum1 : Sum  Inputs=|++
  abc : Outport
  wires:
  Saturation/1 -> abc/1
  Discrete-Time Integrator/1 -> Sum1/2
  Sum1/1 -> Saturation/1
  Gain/1 -> Sum1/1
  Gain1/1 -> Discrete-Time Integrator/1
  Sum/1 -> Gain/1, Gain1/1
  meas/1 -> Sum/2
  ref/1 -> Sum/1

== system Wind_turbine_model_L/Generator/Controller/Subsystem ==
  Vs : Inport
  tita_m : Inport  Port=2
  Atan2 : Trigonometry  Operator=atan2
  Constant : Constant  Value=pi/2
  D/Q-->alfa/beta : Subsystem
  Demux : Demux  Outputs=2
  Gain : Gain  Gain=p
  Sum : Sum  Inputs=|+-
  Sum1 : Sum  Inputs=|+-
  tita_r : Outport
  wires:
  Gain/1 -> Sum1/2
  Sum1/1 -> tita_r/1  "tita_s"
  tita_m/1 -> Gain/1
  Sum/1 -> Sum1/1
  Constant/1 -> Sum/2
  Atan2/1 -> Sum/1
  Demux/2 -> Atan2/1
  Demux/1 -> Atan2/2
  D/Q-->alfa/beta/1(alfa/beta) -> Demux/1
  Vs/1 -> D/Q-->alfa/beta/1(abc)

== system Wind_turbine_model_L/Generator/Controller/abc-->D//Q ==
  abc : Inport
  Fcn : Fcn  Expr=2/3*(u[1]-u[2]/2-u[3]/2)
  Fcn1 : Fcn  Expr=2/3*(u[2]*(sqrt(3)/2)-u[3]*(sqrt(3)/2))
  Mux : Mux  Inputs=2
  D/Q : Outport
  wires:
  Mux/1 -> D/Q/1
  Fcn1/1 -> Mux/2
  Fcn/1 -> Mux/1
  abc/1 -> Fcn/1, Fcn1/1

== system Wind_turbine_model_L/Generator/Controller/d//q-->D//Q ==
  d/q : Inport
  tita : Inport  Port=2
  Fcn : Fcn  Expr=u[1]*cos(u[3])-u[2]*sin(u[3])
  Fcn1 : Fcn  Expr=u[1]*sin(u[3])+u[2]*cos(u[3])
  Mux : Mux  Inputs=2
  Mux1 : Mux  Inputs=2
  D/Q : Outport
  wires:
  Mux1/1 -> Fcn1/1, Fcn/1
  tita/1 -> Mux1/2
  d/q/1 -> Mux1/1
  Mux/1 -> D/Q/1
  Fcn1/1 -> Mux/2
  Fcn/1 -> Mux/1

== system Wind_turbine_model_L/Pitch_Controller/Controller/Ke ==
  ey : Inport
  Gain : Gain  Gain=Tpe
  Gain1 : Gain  Gain=Tie
  Gain2 : Gain  Gain=sigma
  Integrator : Integrator
  Product : Product
  Subtract : Sum
  Subtract1 : Sum  Inputs=+-
  Ke : Outport
  wires:
  Subtract/1 -> Ke/1
  ey/1 -> Product/2, Product/1
  Product/1 -> Gain1/1, Gain/1
  Gain/1 -> Subtract/1
  Gain1/1 -> Subtract1/1
  Subtract1/1 -> Integrator/1
  Integrator/1 -> Gain2/1, Subtract/2
  Gain2/1 -> Subtract1/2

== system Wind_turbine_model_L/Pitch_Controller/Controller/Ku ==
  ey : Inport
  um : Inport  Port=2
  Gain : Gain  Gain=Tpu
  Gain1 : Gain  Gain=Tiu
  Gain2 : Gain  Gain=sigma
  Integrator : Integrator
  Product : Product
  Subtract : Sum
  Subtract1 : Sum  Inputs=+-
  Ku : Outport
  wires:
  Gain2/1 -> Subtract1/2
  Integrator/1 -> Subtract/2, Gain2/1
  Subtract1/1 -> Integrator/1
  Gain1/1 -> Subtract1/1
  Gain/1 -> Subtract/1
  Product/1 -> Gain/1, Gain1/1
  Subtract/1 -> Ku/1
  ey/1 -> Product/1
  um/1 -> Product/2

== system Wind_turbine_model_L/Pitch_Controller/Controller/Kx ==
  ey : Inport
  xm : Inport  Port=2
  Gain : Gain  Gain=Tpx
  Gain1 : Gain  Gain=Tix
  Gain2 : Gain  Gain=sigma
  Integrator : Integrator
  Product : Product
  Subtract : Sum
  Subtract1 : Sum  Inputs=+-
  Kx : Outport
  wires:
  Subtract/1 -> Kx/1
  Gain/1 -> Subtract/1
  Gain1/1 -> Subtract1/1
  Subtract1/1 -> Integrator/1
  Integrator/1 -> Gain2/1, Subtract/2
  Gain2/1 -> Subtract1/2
  Product/1 -> Gain1/1, Gain/1
  ey/1 -> Product/1
  xm/1 -> Product/2

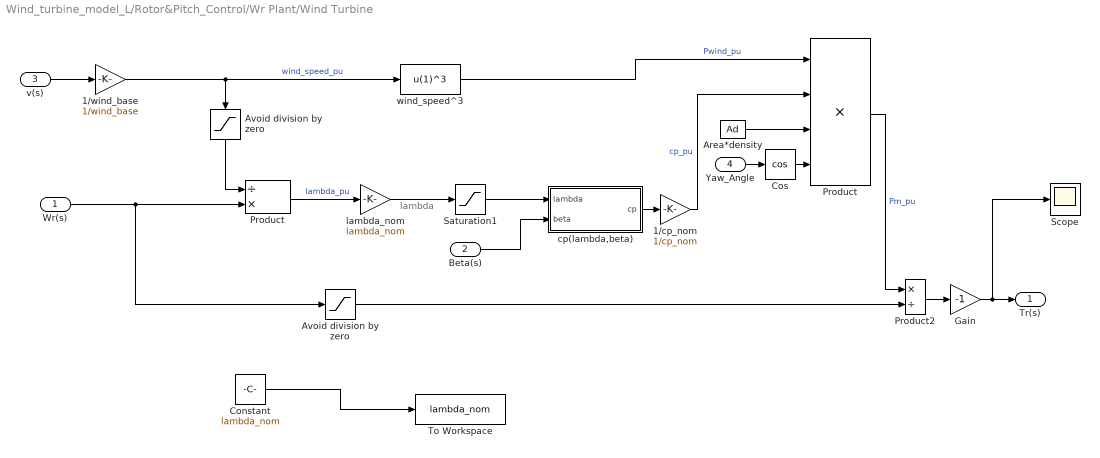
== system Wind_turbine_model_L/Rotor&Pitch_Control/Wr Plant/Wind Turbine ==
  note: lambda
  Wr(s) : Inport
  Beta(s) : Inport  Port=2
  v(s) : Inport  Port=3
  Yaw_Angle : Inport  Port=4
  1/cp_nom : Gain  Gain=1/cp_nom  SaturateOnIntegerOverflow=on  OutDataTypeStr=Inherit: Same as input  ParamDataTypeStr=Inherit: Same as input
  1/wind_base : Gain  Gain=1/wind_base  SaturateOnIntegerOverflow=on  OutDataTypeStr=Inherit: Same as input  ParamDataTypeStr=Inherit: Same as input
  Area*density : Constant  Value=Ad
  Avoid division by zero : Saturate  UpperLimit=1e6  LowerLimit=1e-6
  "Avoid division by zero " : Saturate  UpperLimit=1e6  LowerLimit=1e-6
  Constant : Constant  Value=lambda_nom
  Cos : Trigonometry  Operator=cos
  Gain : Gain  Gain=-1  SaturateOnIntegerOverflow=on  OutDataTypeStr=Inherit: Same as input  ParamDataTypeStr=Inherit: Same as input
  Product : Product  Inputs=/*  SaturateOnIntegerOverflow=on  OutDataTypeStr=Inherit: Same as first input
  "Product " : Product  Inputs=4  SaturateOnIntegerOverflow=on  OutDataTypeStr=Inherit: Same as first input
  Product2 : Product  Inputs=*/  InputSameDT=on  SaturateOnIntegerOverflow=on  OutDataTypeStr=Inherit: Same as first input
  Saturation1 : Saturate  UpperLimit=inf  LowerLimit=1e-6
  Scope : Scope
  To Workspace : ToWorkspace  VariableName=lambda_nom  SaveFormat=Timeseries  SampleTime=-1
  cp(lambda,beta) : Subsystem
  lambda_nom : Gain  Gain=lambda_nom  SaturateOnIntegerOverflow=on  OutDataTypeStr=Inherit: Same as input  ParamDataTypeStr=Inherit: Same as input
  wind_speed^3 : Fcn  Expr=u(1)^3
  Tr(s) : Outport
  wires:
  Area*density/1 -> "Product "/3
  Wr(s)/1 -> Avoid division by zero/1, Product/2
  "Avoid division by zero "/1 -> Product/1
  1/wind_base/1 -> "Avoid division by zero "/1, wind_speed^3/1  "wind_speed_pu"
  Product/1 -> lambda_nom/1  "lambda_pu"
  Saturation1/1 -> cp(lambda,beta)/1(lambda)
  1/cp_nom/1 -> "Product "/2  "cp_pu"
  lambda_nom/1 -> Saturation1/1
  "Product "/1 -> Product2/1  "Pm_pu"
  v(s)/1 -> 1/wind_base/1
  Avoid division by zero/1 -> Product2/2
  Product2/1 -> Gain/1
  wind_speed^3/1 -> "Product "/1  "Pwind_pu"
  cp(lambda,beta)/1(cp) -> 1/cp_nom/1
  Beta(s)/1 -> cp(lambda,beta)/2(beta)
  Gain/1 -> Scope/1, Tr(s)/1
  Constant/1 -> To Workspace/1
  Yaw_Angle/1 -> Cos/1
  Cos/1 -> "Product "/4

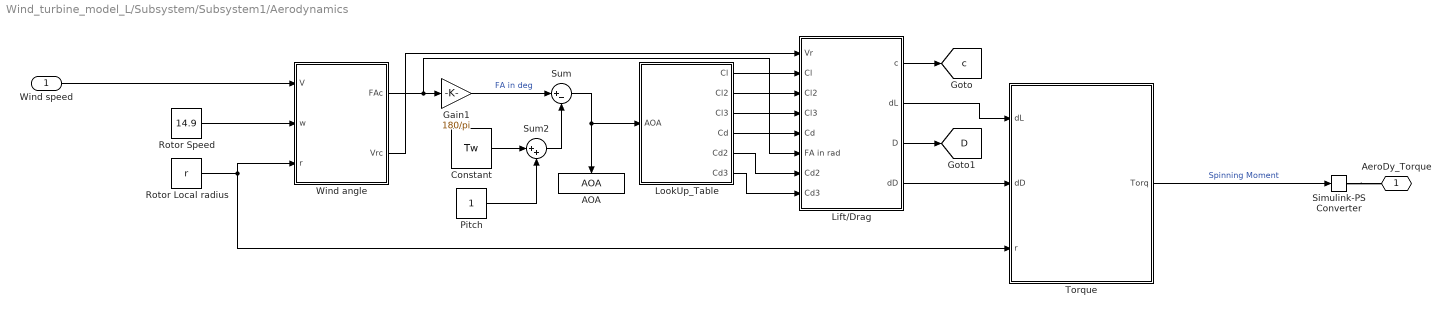
== system Wind_turbine_model_L/Subsystem/Subsystem1/Aerodynamics ==
  Wind speed : Inport
  AOA : ToWorkspace  VariableName=AOA  SampleTime=-1
      settings: Save2DSignal=2-D array (concatenate along first dimension)
  Constant : Constant  Value=Tw  VectorParams1D=off  SampleTime=-1
  Gain1 : Gain  Gain=180/pi
  Lift/Drag : Subsystem
  LookUp_Table : Subsystem
  Pitch : Constant
  Rotor Local radius : Constant  Value=r
  Rotor Speed : Constant  Value=14.9  VectorParams1D=off
  Simulink-PS Converter : nesl_utility/Simulink-PS Converter  PhysicalDomain=network_engine_domain  SubClassName=ps_input  LeftPortType=input  RightPortType=output  PseudoPeriodic=off  Frequencies=[]  NoiseDistribution=none  NoiseParameters=[]  Unit=1  AffineConversion=off  FilteringAndDerivatives=provide  SimscapeFilterOrder=1  InputFilterTimeConstant=0.001  UdotUserProvided=0
  Sum : Sum  Inputs=|+-
  Sum2 : Sum  Inputs=|++
  Torque : Subsystem
  Wind angle : Subsystem
  AeroDy_Torque : PMIOPort  Side=Right
  tag scope: D=global, c=global
  wires:
  Rotor Local radius/1 -> Torque/3(r), Wind angle/3(r)
  Sum/1 -> LookUp_Table/1(AOA), AOA/1
  Lift/Drag/1(c) -> [c]
  Lift/Drag/3(D) -> [D]
  LookUp_Table/1(Cl) -> Lift/Drag/2(Cl)
  LookUp_Table/4(Cd) -> Lift/Drag/5(Cd)
  LookUp_Table/3(Cl3) -> Lift/Drag/4(Cl3)
  LookUp_Table/2(Cl2) -> Lift/Drag/3(Cl2)
  Lift/Drag/2(dL) -> Torque/1(dL)
  Pitch/1 -> Sum2/2
  Wind angle/2(Vrc) -> Lift/Drag/1(Vr)
  Constant/1 -> Sum2/1
  Sum2/1 -> Sum/2
  LookUp_Table/6(Cd3) -> Lift/Drag/8(Cd3)
  Torque/1(Torq) -> Simulink-PS Converter/1  "Spinning Moment"
  Lift/Drag/4(dD) -> Torque/2(dD)
  Wind angle/1(FAc) -> Lift/Drag/6(FA in rad), Gain1/1
  Rotor Speed/1 -> Wind angle/2(w)
  LookUp_Table/5(Cd2) -> Lift/Drag/7(Cd2)
  Gain1/1 -> Sum/1  "FA in deg"
  Wind speed/1 -> Wind angle/1(V)
  connections:
  Simulink-PS Converter/RConn1 -- AeroDy_Torque/RConn1
